simulink model "EEBL_Scenario_03_cs"  (Simulink 7.6)
settings: Solver=ode5  SolverMode=SingleTasking  StartTime=0.0  StopTime=15  FixedStep=1/100  RelTol=1e-3
PreLoadFcn:
  | check_NUTS_defined;
  | 
  | assignin('base',['model_closed_' bdroot],false);addpath('../includes_V2x');
InitFcn:
  | PreScanExperimentInitFcn(bdroot)
StopFcn:
  | PreScanExperimentStopFcn(bdroot)
undefined symbols (not defined in the file): acceleration, actorID, actorType, DiscIntNeverNeededParam, GPS_alt, GPS_lat, GPS_long, intmax, lightBarInUse, messageID, publicVehicleType, rotZ, sireneInUse, trafficLightPriority, turnAdvice, velocity, x_ini_VRML, y_ini_VRML, yawRate, z_ini_VRML
libraries: simulink x68, PreScanSimulinkLibrary x15, simulink_extras x9, PreScanUsefulBlocks x8, simulink_need_slupdate x1
(part 9 of 12)

== system EEBL_Scenario_03_cs/Audi_A8_1/Dynamics_Simple/ShiftLogic ==
  Throttle_[%] : Inport
  GearNr_[-] : Inport  Port=2
  Auto_GearShift : Inport  Port=3
  VehSpeed_[ms-1] : Inport  Port=4
  Add2 : Sum
  Data Type Conversion1 : DataTypeConversion  OutDataTypeStr=double
  Detect Increase1 : simulink/Logic and Bit Operations/Detect Increase  SystemSampleTime=-1  vinit=0.0
  Detect Increase : Subsystem
  Gear limitation : Saturate  UpperLimit=p.maxGear  LowerLimit=1
  Gear limitation while shifting : Saturate  UpperLimit=p.maxGear  LowerLimit=1
  GearNeutral : Constant  Value=0
  GearReverse : Constant  Value=-1
  "IC, gear = 1" : Memory  X0=1  InheritSampleTime=on
  If Action Neutral : Subsystem  TreatAsAtomicUnit=on
  If Action Normal : Subsystem  TreatAsAtomicUnit=on
  If Action Reverse : Subsystem  TreatAsAtomicUnit=on
  Memory : Memory  InheritSampleTime=on
  Merge : Merge  Inputs=3
  Relational Operator : RelationalOperator  OutDataTypeStr=boolean
  Relational Operator1 : RelationalOperator  Operator=<=  OutDataTypeStr=boolean
  Shift_Down time : simulink/Discrete/Integer Delay  NumDelays=p.ShiftDown_fac  InputProcessing=Inherited  vinit=0.0  samptime=-1
  Shift_Up time : simulink/Discrete/Integer Delay  NumDelays=p.ShiftUp_fac  InputProcessing=Inherited  vinit=0.0  samptime=-1
  Sum : Sum  Inputs=+-
  interp_down : Lookup2D  RowIndex=p.downth  ColumnIndex=[1:p.maxGear]  Table=p.downtab  LookUpMeth=Interpolation-Use End Values  InputSameDT=on
  interp_up : Lookup2D  RowIndex=p.upth  ColumnIndex=[1:p.maxGear]  Table=p.uptab  LookUpMeth=Interpolation-Use End Values  InputSameDT=on
  reverse/neutral/normal gear : If  IfExpression=u1 == 0  ElseIfExpressions=u1 < 0
  to_ms-1 : Gain  Gain=1/3.6
  "to_ms-1 " : Gain  Gain=1/3.6
  GearNr : Outport
  wires:
  Auto_GearShift/1 -> reverse/neutral/normal gear/1
  "IC, gear = 1"/1 -> If Action Normal/1(In1)
  Merge/1 -> GearNr/1
  If Action Reverse/1(Out1) -> Merge/2
  If Action Neutral/1(Out1) -> Merge/1
  If Action Normal/1(Out1) -> Merge/3
  reverse/neutral/normal gear/3 -> If Action Normal/Action
  reverse/neutral/normal gear/1 -> If Action Neutral/Action
  reverse/neutral/normal gear/2 -> If Action Reverse/Action
  GearReverse/1 -> If Action Reverse/1(In1)
  GearNeutral/1 -> If Action Neutral/1(In1)
  Shift_Down time/1 -> Sum/2
  Shift_Up time/1 -> Sum/1
  Detect Increase/1(Out1) -> Shift_Up time/1
  Data Type Conversion1/1 -> Shift_Down time/1
  Detect Increase1/1 -> Data Type Conversion1/1
  Sum/1 -> Add2/1
  Memory/1 -> Add2/2  "GearNr_[-]"
  Add2/1 -> Gear limitation while shifting/1
  Gear limitation while shifting/1 -> "IC, gear = 1"/1, Memory/1  "GearNr_[-]"
  Throttle_[%]/1 -> interp_down/1, interp_up/1
  Relational Operator/1 -> Detect Increase/2(In2)
  Relational Operator1/1 -> Detect Increase1/1
  interp_down/1 -> "to_ms-1 "/1
  VehSpeed_[ms-1]/1 -> Relational Operator/1, Relational Operator1/1
  interp_up/1 -> to_ms-1/1
  Gear limitation/1 -> interp_down/2, interp_up/2, Detect Increase/1(GearNr_[-])
  GearNr_[-]/1 -> Gear limitation/1
  to_ms-1/1 -> Relational Operator/2
  "to_ms-1 "/1 -> Relational Operator1/2

== system EEBL_Scenario_03_cs/Audi_A8_1/Dynamics_Simple/Transmission ==
  nEngine_[rpm] : Inport
  GearNr_[-] : Inport  Port=2
  n_TransmissionOut_[rpm] : Inport  Port=3
  Torque_Converter : Subsystem
      mask Display: image(imread('TorqueConverter.png'));
  Transmission_Ratio : Subsystem
  Viscous coupling : Lookup  InputValues=[-5:0.1:5]*p.m/4  Table=p.m/4*tanh([-5:0.1:5])
  ImpellerTorque_[Nm] : Outport  InitialOutput=0
  TransmissionTorque_[Nm] : Outport  Port=2  InitialOutput=0
  wires:
  Torque_Converter/2(TurbineTorque_[Nm]) -> Viscous coupling/1  "Converter_Torque_[Nm]"
  Transmission_Ratio/2(nTransmissionIn_[rpm]) -> Torque_Converter/2(nTransmission_[rpm])
  nEngine_[rpm]/1 -> Torque_Converter/1(nEngine_[rpm])
  GearNr_[-]/1 -> Transmission_Ratio/2(GearNr_[-]), Torque_Converter/3(Gear nr)
  n_TransmissionOut_[rpm]/1 -> Transmission_Ratio/3(nTransmissionOut_[rpm])
  Torque_Converter/1(ImpellerTorque_[Nm]) -> ImpellerTorque_[Nm]/1
  Transmission_Ratio/1(tTransmissionOut_[Nm]) -> TransmissionTorque_[Nm]/1
  Viscous coupling/1 -> Transmission_Ratio/1(tTransmissionIn_[Nm])

== system EEBL_Scenario_03_cs/Audi_A8_1/EEB/vehicle CAM generator ==
  note: System creates continous signals based on CAM protocol
  CAM_warning_in : Inport
  CAM_messageID_in : Inport  Port=2
  CAM_vehicleID_in : Inport  Port=3
  CAM_vehicleType_in : Inport  Port=4
  CAM_publicVehicleType_in : Inport  Port=5
  CAM_lightBarInUse_in : Inport  Port=6
  CAM_sireneInUse_in : Inport  Port=7
  CAM_velocity_in : Inport  Port=8
  CAM_acceleration_in : Inport  Port=9
  CAM_yawRate_in : Inport  Port=10
  CAM_turnAdvice_in : Inport  Port=11
  CAM_trafficLightPriority_in : Inport  Port=12
  CAM_GPSlat_in : Inport  Port=13
  CAM_GPSlong_in : Inport  Port=14
  CAM_GPSalt_in : Inport  Port=15
  CAM_rotZ_in : Inport  Port=16
  NoMissedMessages : Inport  Port=17
  MessageDelay : Inport  Port=18
  CAM delay : Subsystem
  For Iterator Subsystem : Subsystem  TreatAsAtomicUnit=on
  Memory : Memory
  Memory1 : Memory
  Probe : Probe  ProbeWidth=off  ProbeSampleTime=off  ProbeComplexSignal=off  ProbeSignalDimensions=on
  Rounding Function1 : Rounding
  Seperate signals : Stateflow chart  TreatAsAtomicUnit=on
  Signal Matrix create : Stateflow chart  TreatAsAtomicUnit=on
  CAM_warning : Outport
  CAM_messageID : Outport  Port=2
  CAM_vehicleID : Outport  Port=3
  CAM_vehicleType : Outport  Port=4
  CAM_publicVehicleType : Outport  Port=5
  CAM_lightBarInUse : Outport  Port=6
  CAM_sireneInUse : Outport  Port=7
  CAM_velocity : Outport  Port=8
  CAM_acceleration : Outport  Port=9
  CAM_yawRate : Outport  Port=10
  CAM_turnAdvice : Outport  Port=11
  CAM_trafficLightPriority : Outport  Port=12
  CAM_GPSlat : Outport  Port=13
  CAM_GPSlong : Outport  Port=14
  CAM_GPSalt : Outport  Port=15
  CAM_rotZ : Outport  Port=16
  wires:
  Seperate signals/16(CAM_rotZ) -> CAM_rotZ/1
  Seperate signals/15(CAM_GPSalt) -> CAM_GPSalt/1
  Seperate signals/14(CAM_GPSlong) -> CAM_GPSlong/1
  Seperate signals/13(CAM_GPSlat) -> CAM_GPSlat/1
  Seperate signals/12(CAM_trafficLightPriority) -> CAM_trafficLightPriority/1
  Seperate signals/11(CAM_turnAdvice) -> CAM_turnAdvice/1
  Seperate signals/10(CAM_yawRate) -> CAM_yawRate/1
  Seperate signals/9(CAM_acceleration) -> CAM_acceleration/1
  Seperate signals/8(CAM_velocity) -> CAM_velocity/1
  Seperate signals/7(CAM_sireneInUse) -> CAM_sireneInUse/1
  Seperate signals/6(CAM_lightBarInUse) -> CAM_lightBarInUse/1
  Seperate signals/5(CAM_publicVehicleType) -> CAM_publicVehicleType/1
  Seperate signals/4(CAM_vehicleType) -> CAM_vehicleType/1
  Seperate signals/3(CAM_vehicleID) -> CAM_vehicleID/1
  Seperate signals/2(CAM_messageID) -> CAM_messageID/1
  Seperate signals/1(CAM_warning) -> CAM_warning/1
  CAM_warning_in/1 -> Signal Matrix create/1(CAM_warning)
  CAM_messageID_in/1 -> Signal Matrix create/2(CAM_messageID)
  CAM_vehicleID_in/1 -> Signal Matrix create/3(CAM_vehicleID), Probe/1
  CAM_vehicleType_in/1 -> Signal Matrix create/4(CAM_vehicleType)
  CAM_publicVehicleType_in/1 -> Signal Matrix create/5(CAM_publicVehicleType)
  CAM_lightBarInUse_in/1 -> Signal Matrix create/6(CAM_lightBarInUse)
  CAM_sireneInUse_in/1 -> Signal Matrix create/7(CAM_sireneInUse)
  CAM_velocity_in/1 -> Signal Matrix create/8(CAM_velocity)
  CAM_acceleration_in/1 -> Signal Matrix create/9(CAM_acceleration)
  CAM_yawRate_in/1 -> Signal Matrix create/10(CAM_yawRate)
  CAM_turnAdvice_in/1 -> Signal Matrix create/11(CAM_turnAdvice)
  CAM_trafficLightPriority_in/1 -> Signal Matrix create/12(CAM_trafficLightPriority)
  CAM_GPSlat_in/1 -> Signal Matrix create/13(CAM_GPSlat)
  CAM_GPSlong_in/1 -> Signal Matrix create/14(CAM_GPSlong)
  CAM_GPSalt_in/1 -> Signal Matrix create/15(CAM_GPSalt)
  CAM_rotZ_in/1 -> Signal Matrix create/16(CAM_rotZ)
  Memory/1 -> For Iterator Subsystem/3(CAM_old)
  For Iterator Subsystem/1(CAM_o) -> Memory/1, Seperate signals/1(CAM)
  Probe/1 -> For Iterator Subsystem/2(Size)
  Signal Matrix create/1(CAM) -> CAM delay/1(in)
  MessageDelay/1 -> CAM delay/2(Tdelay)
  CAM delay/1(out) -> For Iterator Subsystem/1(CAM_in)
  For Iterator Subsystem/2(tmp_out) -> Memory1/1
  Memory1/1 -> For Iterator Subsystem/5(tmp_in)
  NoMissedMessages/1 -> Rounding Function1/1
  Rounding Function1/1 -> For Iterator Subsystem/4(NoMM)

== system EEBL_Scenario_03_cs/Audi_A8_1/PathFollower_1/CTRL REFERENCES ==
  note: REFERENCE POSITION BASED POSITION CTRL
  Pos x,y,Y [m,m,rad] : Inport
  Position Preview Distance [m] : Inport  Port=2
  TrajOffset [m,m,rad] : Inport  Port=3
  ActorOffset_Left(+) / Right(-)_[m] : Inport  Port=4
  Calculate Preview Point (pvp) by extrapolating current Vehicle Position (p0) with Preview Distance and Vehicle Orientation : Subsystem
  Find Reference Point (pref)  on Trajectory closest  to PreView Point (pvp) : M-S-Function  FunctionName=msfcn_find_closest_trajectory_points  Parameters=[Traj_x Traj_y]
      mask Display:
      | port_label('input', 1, 'pvp')
      | port_label('input', 2, 'TrajOffset_x_y_Y')
      | port_label('input', 3, 'ActorOffset_Left+/Right-')
      | port_label('input', 4, 'p0')
      | port_label('output', 1, 'pref')
  Find Reference Point (pref0)  on Trajectory closest  to P0 Point (p0) : M-S-Function  FunctionName=msfcn_find_closest_trajectory_points0  Parameters=[Traj_x Traj_y]
      mask Display:
      | port_label('input', 1, 'pvp')
      | port_label('input', 2, 'TrajOffset_x_y_Y')
      | port_label('input', 3, 'ActorOffset_Left+/Right-')
      | port_label('input', 4, 'p0')
      | port_label('output', 1, 'pref_0')
      | port_label('output', 2, 'Actor/Traj_distance')
      | port_label('output', 3, 'Actor/Traj_angle')
  Mux1 : Mux  Inputs=2
  Selector1 : Selector  InputPortWidth=3  IndexOptions=Index vector (dialog)  Indices=[1 2]  OutputSizes=1
  Terminator : Terminator
  pvp  [m,m] : Outport
  pref_pvp [m,m] : Outport  Port=2
  pref_0 [m,m] : Outport  Port=3
  Actor/Traj_distance [m] : Outport  Port=4
  Actor/Traj_angle [deg] : Outport  Port=5
  wires:
  Mux1/1 -> pvp  [m,m]/1, Find Reference Point (pref)  on Trajectory closest  to PreView Point (pvp)/1, Find Reference Point (pref0)  on Trajectory closest  to P0 Point (p0)/1
  Pos x,y,Y [m,m,rad]/1 -> Calculate Preview Point (pvp) by extrapolating current Vehicle Position (p0) with Preview Distance and Vehicle Orientation/2(x,y,Y Demux [m,m,rad]), Find Reference Point (pref0)  on Trajectory closest  to P0 Point (p0)/4, Selector1/1
  Calculate Preview Point (pvp) by extrapolating current Vehicle Position (p0) with Preview Distance and Vehicle Orientation/1(x_glob_PVD) -> Mux1/1
  Calculate Preview Point (pvp) by extrapolating current Vehicle Position (p0) with Preview Distance and Vehicle Orientation/3(Y [rad]) -> Terminator/1
  Position Preview Distance [m]/1 -> Calculate Preview Point (pvp) by extrapolating current Vehicle Position (p0) with Preview Distance and Vehicle Orientation/1(Preview Distance)
  Find Reference Point (pref)  on Trajectory closest  to PreView Point (pvp)/1 -> pref_pvp [m,m]/1
  Find Reference Point (pref0)  on Trajectory closest  to P0 Point (p0)/1 -> pref_0 [m,m]/1
  Calculate Preview Point (pvp) by extrapolating current Vehicle Position (p0) with Preview Distance and Vehicle Orientation/2(y_glob_PVD) -> Mux1/2
  TrajOffset [m,m,rad]/1 -> Find Reference Point (pref)  on Trajectory closest  to PreView Point (pvp)/2, Find Reference Point (pref0)  on Trajectory closest  to P0 Point (p0)/2  "L6"
  ActorOffset_Left(+) / Right(-)_[m]/1 -> Find Reference Point (pref)  on Trajectory closest  to PreView Point (pvp)/3, Find Reference Point (pref0)  on Trajectory closest  to P0 Point (p0)/3
  Selector1/1 -> Find Reference Point (pref)  on Trajectory closest  to PreView Point (pvp)/4
  Find Reference Point (pref0)  on Trajectory closest  to P0 Point (p0)/2 -> Actor/Traj_distance [m]/1
  Find Reference Point (pref0)  on Trajectory closest  to P0 Point (p0)/3 -> Actor/Traj_angle [deg]/1

== system EEBL_Scenario_03_cs/Audi_A8_1/PathFollower_1/Calculate shifted p0 wrt COG ==
  position x,y,Y [m,m,deg] : Inport
  Constant1 : Constant  Value=XShifting_wrt_COG
  Degrees to Radians : simulink_extras/Transformations/Degrees to Radians  SystemSampleTime=-1
  Demux1 : Demux  Outputs=3
  Fcn : Fcn  Expr=u(2)*cos(u(1))
  Fcn1 : Fcn  Expr=u(2)*sin(u(1))
  Mux1 : Mux  Inputs=3
  Mux2 : Mux  Inputs=2
  Sum : Sum  Inputs=|++
  Sum1 : Sum  Inputs=|++
  position x,y,Y [m,m,rad] : Outport
  wires:
  Sum/1 -> Mux1/1
  Sum1/1 -> Mux1/2
  Demux1/1 -> Sum/1
  Demux1/3 -> Degrees to Radians/1
  Degrees to Radians/1 -> Mux2/1, Mux1/3
  Mux2/1 -> Fcn/1, Fcn1/1
  Fcn/1 -> Sum/2
  Fcn1/1 -> Sum1/2
  Demux1/2 -> Sum1/1
  position x,y,Y [m,m,deg]/1 -> Demux1/1
  Mux1/1 -> position x,y,Y [m,m,rad]/1
  Constant1/1 -> Mux2/2

== system EEBL_Scenario_03_cs/Audi_A8_1/PathFollower_1/DELTA CTRL ==
  note: POSITION BASED STEERWHEEL CONTROL
  p0 : Inport
  pvp : Inport  Port=2
  pref_pvp : Inport  Port=3
  pref0 : Inport  Port=4
  Calculate  preview angle : M-S-Function  FunctionName=msfcn_preview_angle_and_distance
      mask Display:
      | port_label('input', 2, 'pref [m,m]')
      | port_label('input', 3, 'p0 [m,m]')
      | port_label('input', 1, 'pvp [m,m]')
      | 
      | port_label('output', 1, 'angle [rad]')
  Divide2 : Product
  Divide4 : Product
  Error check : Subsystem
  Goto Tag Visibility : GotoTagVisibility  GotoTag=pref0
  Goto Tag Visibility1 : GotoTagVisibility  GotoTag=p0
  Radians to Degrees1 : simulink_extras/Transformations/Radians to Degrees  SystemSampleTime=-1
  Selector2 : Selector  InputPortWidth=3  IndexOptions=Index vector (dialog)  Indices=[1 2]  OutputSizes=1
  Steering angle  velocity dependent : Lookup  InputValues=[0 18 40 60 70 80 90 100 110]  Table=[16.5 16.5 28 44.5 55 60.5 60.5 60.5 60.5]
  Steering angle preview  distance dependent : Lookup  InputValues=[0 1 4 5 6 7 8 9 10 11 20 21]  Table=[1.5 1.5 1 1 1 1 1 1 0.9 0.9 0.8 0.8]
  These limits are  the vehicle maximum  steering wheel angle : Saturate  UpperLimit=720  LowerLimit=-720
  TunableSteering Gain : Gain  Gain=TunableSteeringGain
  sign1 : Gain  Gain=3.6
  delta_steerwheel [deg] : Outport
  tag scope: p0=scoped, pref0=scoped
  wires:
  Calculate  preview angle/1 -> Radians to Degrees1/1
  Selector2/1 -> Calculate  preview angle/3
  p0/1 -> Selector2/1, [p0]
  pvp/1 -> Calculate  preview angle/1
  pref_pvp/1 -> Calculate  preview angle/2
  Radians to Degrees1/1 -> Divide2/2
  These limits are  the vehicle maximum  steering wheel angle/1 -> delta_steerwheel [deg]/1
  pref0/1 -> [pref0]
  sign1/1 -> Steering angle  velocity dependent/1
  [v_actual] -> sign1/1
  Steering angle  velocity dependent/1 -> Divide2/1
  Divide4/1 -> TunableSteering Gain/1
  Divide2/1 -> Divide4/1
  Steering angle preview  distance dependent/1 -> Divide4/2
  [PreviewDistance] -> Steering angle preview  distance dependent/1
  TunableSteering Gain/1 -> These limits are  the vehicle maximum  steering wheel angle/1

== system EEBL_Scenario_03_cs/Audi_A8_1/PathFollower_1/THROTTLE CTRL ==
  v_actual [m/s] : Inport
  Desired Velocity [m/s] : Inport  Port=2
  Initial Velocity [m/s] : Inport  Port=3
  Demux : Demux  Outputs=3
  GearNormal : Constant
  "GearNormal " : Constant
  If Desired Velocity = 0 : Subsystem  TreatAsAtomicUnit=on
  If Desired Velocity ~= 0 : Subsystem  TreatAsAtomicUnit=on
  Merge : Merge
  Mux : Mux  Inputs=3
  Mux2 : Mux  Inputs=3
  Sum4 : Sum  Inputs=|+-
  if : If  IfExpression=u1 == 0
  throttle [%] : Outport
  brake pressure [bar] : Outport  Port=2
  v0 [m/s] : Outport  Port=3
  Auto_GearShift : Outport  Port=4
  wires:
  v_actual [m/s]/1 -> Sum4/2
  If Desired Velocity ~= 0/3(Auto_GearShift) -> Mux2/3
  If Desired Velocity ~= 0/2(brake pressure [bar]) -> Mux2/2
  If Desired Velocity ~= 0/1(throttle [%]) -> Mux2/1
  if/1 -> If Desired Velocity = 0/Action
  if/2 -> If Desired Velocity ~= 0/Action
  If Desired Velocity = 0/3(Auto_GearShift) -> Mux/3
  "GearNormal "/1 -> If Desired Velocity ~= 0/1(In1)
  Demux/3 -> Auto_GearShift/1
  Demux/2 -> brake pressure [bar]/1
  Demux/1 -> throttle [%]/1
  Mux/1 -> Merge/1
  Mux2/1 -> Merge/2
  If Desired Velocity = 0/2(brake pressure [bar]) -> Mux/2
  If Desired Velocity = 0/1(throttle [%]) -> Mux/1
  Merge/1 -> Demux/1
  GearNormal/1 -> If Desired Velocity = 0/1(In1)
  Initial Velocity [m/s]/1 -> v0 [m/s]/1
  Desired Velocity [m/s]/1 -> Sum4/1, if/1
  Sum4/1 -> If Desired Velocity ~= 0/2(Desired Velocity [m/s])

== system EEBL_Scenario_03_cs/Audi_A8_1/SELF_Demux/compas converter ==
  rotz [rad] : Inport
  cart2compas : Subsystem
  rad2deg : Gain  Gain=180/pi
  heading [deg] : Outport
  wires:
  cart2compas/1(heading [deg]) -> heading [deg]/1
  rotz [rad]/1 -> rad2deg/1
  rad2deg/1 -> cart2compas/1(Angle [deg])

== system EEBL_Scenario_03_cs/Audi_A8_1/Trajectories/Traj2State1 ==
  Traj Org : Inport
  Offset : Inport  Port=2
  Add2 : Sum
  ApplyRotation : PreScanSimulinkLibrary/ApplyRotation  SystemSampleTime=-1
  ApplyRotation1 : PreScanSimulinkLibrary/ApplyRotation  SystemSampleTime=-1
  ApplyRotation2 : PreScanSimulinkLibrary/ApplyRotation  SystemSampleTime=-1
  Constant : Constant  Value=zeros(12,1)
  Mux : Mux  Inputs=6
  Mux1 : Mux  Inputs=2
  Mux{2,4..9} (7 alike) : Mux  Inputs=3
  Mux3 : Mux  Inputs=2
  Selector : Selector  InputPortWidth=6  IndexOptions=Index vector (dialog)  Indices=[4 5 6]  OutputSizes=1
  Selector1 : Selector  InputPortWidth=21  IndexOptions=Index vector (dialog)  Indices=[5]  OutputSizes=1
  Selector10 : Selector  InputPortWidth=21  IndexOptions=Index vector (dialog)  Indices=[2]  OutputSizes=1
  Selector11 : Selector  InputPortWidth=21  IndexOptions=Index vector (dialog)  Indices=[3]  OutputSizes=1
  Selector12 : Selector  InputPortWidth=21  IndexOptions=Index vector (dialog)  Indices=[1]  OutputSizes=1
  Selector13 : Selector  InputPortWidth=21  IndexOptions=Index vector (dialog)  Indices=[8]  OutputSizes=1
  Selector14 : Selector  InputPortWidth=21  IndexOptions=Index vector (dialog)  Indices=[9]  OutputSizes=1
  Selector15 : Selector  InputPortWidth=21  IndexOptions=Index vector (dialog)  Indices=[7]  OutputSizes=1
  Selector16 : Selector  InputPortWidth=21  IndexOptions=Index vector (dialog)  Indices=[14]  OutputSizes=1
  Selector17 : Selector  InputPortWidth=21  IndexOptions=Index vector (dialog)  Indices=[15]  OutputSizes=1
  Selector18 : Selector  InputPortWidth=21  IndexOptions=Index vector (dialog)  Indices=[13]  OutputSizes=1
  Selector19 : Selector  InputPortWidth=21  IndexOptions=Index vector (dialog)  Indices=[20]  OutputSizes=1
  Selector2 : Selector  InputPortWidth=21  IndexOptions=Index vector (dialog)  Indices=[6]  OutputSizes=1
  Selector20 : Selector  InputPortWidth=21  IndexOptions=Index vector (dialog)  Indices=[21]  OutputSizes=1
  Selector21 : Selector  InputPortWidth=21  IndexOptions=Index vector (dialog)  Indices=[19]  OutputSizes=1
  Selector3 : Selector  InputPortWidth=21  IndexOptions=Index vector (dialog)  Indices=[12]  OutputSizes=1
  Selector4 : Selector  InputPortWidth=21  IndexOptions=Index vector (dialog)  Indices=[17]  OutputSizes=1
  Selector5 : Selector  InputPortWidth=21  IndexOptions=Index vector (dialog)  Indices=[18]  OutputSizes=1
  Selector6 : Selector  InputPortWidth=21  IndexOptions=Index vector (dialog)  Indices=[16]  OutputSizes=1
  Selector7 : Selector  InputPortWidth=21  IndexOptions=Index vector (dialog)  Indices=[11]  OutputSizes=1
  Selector8 : Selector  InputPortWidth=21  IndexOptions=Index vector (dialog)  Indices=[10]  OutputSizes=1
  Selector9 : Selector  InputPortWidth=21  IndexOptions=Index vector (dialog)  Indices=[4]  OutputSizes=1
  Traj2State2 : Subsystem
  state : Outport
  wires:
  Mux9/1 -> ApplyRotation2/2, ApplyRotation1/2, ApplyRotation/2
  Selector20/1 -> Mux9/3
  Selector19/1 -> Mux9/2
  Selector21/1 -> Mux9/1
  Selector5/1 -> Mux8/3
  Selector4/1 -> Mux8/2
  Selector6/1 -> Mux8/1
  Mux8/1 -> Mux/6
  Mux6/1 -> ApplyRotation2/1
  Mux7/1 -> Mux/4
  ApplyRotation2/1 -> Mux/5
  Selector3/1 -> Mux7/3
  Selector7/1 -> Mux7/2
  Selector8/1 -> Mux7/1
  Mux4/1 -> Mux/2
  Mux5/1 -> ApplyRotation1/1
  ApplyRotation1/1 -> Mux/3
  Mux2/1 -> ApplyRotation/1
  ApplyRotation/1 -> Mux/1
  Selector2/1 -> Mux4/3
  Selector1/1 -> Mux4/2
  Selector9/1 -> Mux4/1
  Selector17/1 -> Mux6/3
  Selector16/1 -> Mux6/2
  Selector18/1 -> Mux6/1
  Selector14/1 -> Mux5/3
  Selector13/1 -> Mux5/2
  Selector15/1 -> Mux5/1
  Selector11/1 -> Mux2/3
  Selector10/1 -> Mux2/2
  Selector12/1 -> Mux2/1
  Mux3/1 -> Selector8/1, Selector7/1, Selector3/1, Selector18/1, Selector16/1, Selector17/1, Selector6/1, Selector20/1, Selector19/1, Selector21/1, Selector5/1, Selector4/1, Selector14/1, Selector13/1, Selector15/1, Selector2/1, Selector1/1, Selector9/1, Selector12/1, Selector10/1, Selector11/1
  Mux1/1 -> Add2/2
  Constant/1 -> Mux1/2
  Add2/1 -> Traj2State2/1(traj)
  Selector/1 -> Mux3/2
  Traj Org/1 -> Mux3/1
  Offset/1 -> Mux1/1, Selector/1
  Mux/1 -> Add2/1
  Traj2State2/1(state) -> state/1

== system EEBL_Scenario_03_cs/Audi_A8_1/Trajectories/Trajectory_1 ==
  From Workspace : FromWorkspace  VariableName=trajectory  SampleTime=TimeStep  OutputAfterFinalValue=Holding final value
  From Workspace1 : FromWorkspace  VariableName=trajectory  SampleTime=TimeStep  OutputAfterFinalValue=Setting to zero
  Mux : Mux  Inputs=2
  Selector1 : Selector  InputPortWidth=24  IndexOptions=Index vector (dialog)  Indices=[7:18]  OutputSizes=1
  Selector9 : Selector  InputPortWidth=24  IndexOptions=Index vector (dialog)  Indices=[1:6]  OutputSizes=1
  trajectory : Outport
  wires:
  Selector1/1 -> Mux/2
  Selector9/1 -> Mux/1
  Mux/1 -> trajectory/1
  From Workspace1/1 -> Selector1/1
  From Workspace/1 -> Selector9/1

== system EEBL_Scenario_03_cs/BMW_X5_1/Antenna_Rx_3_Demux/Reorder ==
  In : Inport
  Selector1 : Selector  InputPortWidth=InputPortWidth  IndexOptions=Index vector (dialog)  Indices=Elements  OutputSizes=1
  Out : Outport
  wires:
  Selector1/1 -> Out/1
  In/1 -> Selector1/1

== system EEBL_Scenario_03_cs/BMW_X5_1/Antenna_Rx_3_Demux/compas converter ==
  rotz [rad] : Inport
  cart2compas : Subsystem
  rad2deg : Gain  Gain=180/pi
  heading [deg] : Outport
  wires:
  rad2deg/1 -> cart2compas/1(Angle [deg])
  rotz [rad]/1 -> rad2deg/1
  cart2compas/1(heading [deg]) -> heading [deg]/1

== system EEBL_Scenario_03_cs/BMW_X5_1/SELF_Demux/compas converter ==
  rotz [rad] : Inport
  cart2compas : Subsystem
  rad2deg : Gain  Gain=180/pi
  heading [deg] : Outport
  wires:
  cart2compas/1(heading [deg]) -> heading [deg]/1
  rotz [rad]/1 -> rad2deg/1
  rad2deg/1 -> cart2compas/1(Angle [deg])

== system EEBL_Scenario_03_cs/BMW_X5_1/Trajectories/Traj2State1 ==
  Traj Org : Inport
  Offset : Inport  Port=2
  Add2 : Sum
  ApplyRotation : PreScanSimulinkLibrary/ApplyRotation  SystemSampleTime=-1
  ApplyRotation1 : PreScanSimulinkLibrary/ApplyRotation  SystemSampleTime=-1
  ApplyRotation2 : PreScanSimulinkLibrary/ApplyRotation  SystemSampleTime=-1
  Constant : Constant  Value=zeros(12,1)
  Mux : Mux  Inputs=6
  Mux1 : Mux  Inputs=2
  Mux{2,4..9} (7 alike) : Mux  Inputs=3
  Mux3 : Mux  Inputs=2
  Selector : Selector  InputPortWidth=6  IndexOptions=Index vector (dialog)  Indices=[4 5 6]  OutputSizes=1
  Selector1 : Selector  InputPortWidth=21  IndexOptions=Index vector (dialog)  Indices=[5]  OutputSizes=1
  Selector10 : Selector  InputPortWidth=21  IndexOptions=Index vector (dialog)  Indices=[2]  OutputSizes=1
  Selector11 : Selector  InputPortWidth=21  IndexOptions=Index vector (dialog)  Indices=[3]  OutputSizes=1
  Selector12 : Selector  InputPortWidth=21  IndexOptions=Index vector (dialog)  Indices=[1]  OutputSizes=1
  Selector13 : Selector  InputPortWidth=21  IndexOptions=Index vector (dialog)  Indices=[8]  OutputSizes=1
  Selector14 : Selector  InputPortWidth=21  IndexOptions=Index vector (dialog)  Indices=[9]  OutputSizes=1
  Selector15 : Selector  InputPortWidth=21  IndexOptions=Index vector (dialog)  Indices=[7]  OutputSizes=1
  Selector16 : Selector  InputPortWidth=21  IndexOptions=Index vector (dialog)  Indices=[14]  OutputSizes=1
  Selector17 : Selector  InputPortWidth=21  IndexOptions=Index vector (dialog)  Indices=[15]  OutputSizes=1
  Selector18 : Selector  InputPortWidth=21  IndexOptions=Index vector (dialog)  Indices=[13]  OutputSizes=1
  Selector19 : Selector  InputPortWidth=21  IndexOptions=Index vector (dialog)  Indices=[20]  OutputSizes=1
  Selector2 : Selector  InputPortWidth=21  IndexOptions=Index vector (dialog)  Indices=[6]  OutputSizes=1
  Selector20 : Selector  InputPortWidth=21  IndexOptions=Index vector (dialog)  Indices=[21]  OutputSizes=1
  Selector21 : Selector  InputPortWidth=21  IndexOptions=Index vector (dialog)  Indices=[19]  OutputSizes=1
  Selector3 : Selector  InputPortWidth=21  IndexOptions=Index vector (dialog)  Indices=[12]  OutputSizes=1
  Selector4 : Selector  InputPortWidth=21  IndexOptions=Index vector (dialog)  Indices=[17]  OutputSizes=1
  Selector5 : Selector  InputPortWidth=21  IndexOptions=Index vector (dialog)  Indices=[18]  OutputSizes=1
  Selector6 : Selector  InputPortWidth=21  IndexOptions=Index vector (dialog)  Indices=[16]  OutputSizes=1
  Selector7 : Selector  InputPortWidth=21  IndexOptions=Index vector (dialog)  Indices=[11]  OutputSizes=1
  Selector8 : Selector  InputPortWidth=21  IndexOptions=Index vector (dialog)  Indices=[10]  OutputSizes=1
  Selector9 : Selector  InputPortWidth=21  IndexOptions=Index vector (dialog)  Indices=[4]  OutputSizes=1
  Traj2State2 : Subsystem
  state : Outport
  wires:
  Mux9/1 -> ApplyRotation2/2, ApplyRotation1/2, ApplyRotation/2
  Selector20/1 -> Mux9/3
  Selector19/1 -> Mux9/2
  Selector21/1 -> Mux9/1
  Selector5/1 -> Mux8/3
  Selector4/1 -> Mux8/2
  Selector6/1 -> Mux8/1
  Mux8/1 -> Mux/6
  Mux6/1 -> ApplyRotation2/1
  Mux7/1 -> Mux/4
  ApplyRotation2/1 -> Mux/5
  Selector3/1 -> Mux7/3
  Selector7/1 -> Mux7/2
  Selector8/1 -> Mux7/1
  Mux4/1 -> Mux/2
  Mux5/1 -> ApplyRotation1/1
  ApplyRotation1/1 -> Mux/3
  Mux2/1 -> ApplyRotation/1
  ApplyRotation/1 -> Mux/1
  Selector2/1 -> Mux4/3
  Selector1/1 -> Mux4/2
  Selector9/1 -> Mux4/1
  Selector17/1 -> Mux6/3
  Selector16/1 -> Mux6/2
  Selector18/1 -> Mux6/1
  Selector14/1 -> Mux5/3
  Selector13/1 -> Mux5/2
  Selector15/1 -> Mux5/1
  Selector11/1 -> Mux2/3
  Selector10/1 -> Mux2/2
  Selector12/1 -> Mux2/1
  Mux3/1 -> Selector8/1, Selector7/1, Selector3/1, Selector18/1, Selector16/1, Selector17/1, Selector6/1, Selector20/1, Selector19/1, Selector21/1, Selector5/1, Selector4/1, Selector14/1, Selector13/1, Selector15/1, Selector2/1, Selector1/1, Selector9/1, Selector12/1, Selector10/1, Selector11/1
  Mux1/1 -> Add2/2
  Constant/1 -> Mux1/2
  Add2/1 -> Traj2State2/1(traj)
  Selector/1 -> Mux3/2
  Traj Org/1 -> Mux3/1
  Offset/1 -> Mux1/1, Selector/1
  Mux/1 -> Add2/1
  Traj2State2/1(state) -> state/1

== system EEBL_Scenario_03_cs/BMW_X5_1/Trajectories/Trajectory_2 ==
  From Workspace : FromWorkspace  VariableName=trajectory  SampleTime=TimeStep  OutputAfterFinalValue=Holding final value
  From Workspace1 : FromWorkspace  VariableName=trajectory  SampleTime=TimeStep  OutputAfterFinalValue=Setting to zero
  Mux : Mux  Inputs=2
  Selector1 : Selector  InputPortWidth=24  IndexOptions=Index vector (dialog)  Indices=[7:18]  OutputSizes=1
  Selector9 : Selector  InputPortWidth=24  IndexOptions=Index vector (dialog)  Indices=[1:6]  OutputSizes=1
  trajectory : Outport
  wires:
  Selector1/1 -> Mux/2
  Selector9/1 -> Mux/1
  Mux/1 -> trajectory/1
  From Workspace1/1 -> Selector1/1
  From Workspace/1 -> Selector9/1

== system EEBL_Scenario_03_cs/BMW_X5_1/vehicle CAM generator/CAM generation ==
  x [m] : Inport
  y [m] : Inport  Port=2
  z [m] : Inport  Port=3
  rotZ [deg] : Inport  Port=4
  velocity [m/s] : Inport  Port=5
  Enable : EnablePort  StatesWhenEnabling=reset  PropagateVarSize=During execution
  Add : Sum  Inputs=+-
  Data Store Memory : DataStoreMemory  DataStoreName=CAM_time
  Data Store Memory1 : DataStoreMemory  DataStoreName=CAM_velocity
  Data Store Memory2 : DataStoreMemory  DataStoreName=CAM_heading
  Data Store Memory3 : DataStoreMemory  DataStoreName=CAM_x
  Data Store Memory4 : DataStoreMemory  DataStoreName=CAM_y
  Data Store Memory5 : DataStoreMemory  DataStoreName=CAM_z
  Data Store Read : DataStoreRead  DataStoreName=CAM_time  SampleTime=0.01
  Digital Clock : DigitalClock  SampleTime=0.01
  Merge : Merge  Inputs=3
  if : If  IfExpression=u1 >= 1  ElseIfExpressions=u1 < 0.1
  maybe : Subsystem  TreatAsAtomicUnit=on
  no : Subsystem  TreatAsAtomicUnit=on
  yes : Subsystem  TreatAsAtomicUnit=on
  CAN generation signal : Outport  OutputWhenDisabled=reset  InitialOutput=0
  wires:
  Digital Clock/1 -> Add/1
  Data Store Read/1 -> Add/2
  Add/1 -> if/1
  if/1 -> yes/Action
  yes/1(Out1) -> Merge/1
  no/1(Out1) -> Merge/2
  if/2 -> no/Action
  if/3 -> maybe/Action
  Merge/1 -> CAN generation signal/1
  x [m]/1 -> maybe/1(x [m]), yes/1(x [m])
  y [m]/1 -> maybe/2(y [m]), yes/2(y [m])
  z [m]/1 -> maybe/3(z [m]), yes/3(z [m])
  rotZ [deg]/1 -> maybe/4(rotZ [deg]), yes/4(rotZ [deg])
  velocity [m/s]/1 -> maybe/5(velocity [m/s]), yes/5(velocity [m/s])
  maybe/1(Out1) -> Merge/3

== system EEBL_Scenario_03_cs/BMW_X5_1/vehicle CAM generator/Enabled Subsystem ==
  CAM_sig : Inport
  Enable : EnablePort  PropagateVarSize=During execution
  CAM_signals : Outport  OutputWhenDisabled=reset  InitialOutput=0
  wires:
  CAM_sig/1 -> CAM_signals/1

== system EEBL_Scenario_03_cs/BMW_X5_1/vehicle CAM generator/Subsystem ==
  In1 : Inport
  GPS_Noise_src : Inport  Port=2
  GPS Noise : Subsystem
  Sum2 : Sum  Inputs=|++
  Out1 : Outport
  wires:
  GPS Noise/1(GPS_Noise) -> Sum2/2
  In1/1 -> Sum2/1
  Sum2/1 -> Out1/1
  GPS_Noise_src/1 -> GPS Noise/1(GPS_Noise_src)

== system EEBL_Scenario_03_cs/BMW_X5_1/vehicle CAM generator/Subsystem1 ==
  In1 : Inport
  GPS_Noise_src : Inport  Port=2
  GPS Noise : Subsystem
  Sum2 : Sum  Inputs=|++
  Out1 : Outport
  wires:
  GPS_Noise_src/1 -> GPS Noise/1(GPS_Noise_src)
  Sum2/1 -> Out1/1
  In1/1 -> Sum2/1
  GPS Noise/1(GPS_Noise) -> Sum2/2

== system EEBL_Scenario_03_cs/BMW_X5_1/vehicle CAM generator/Subsystem2 ==
  In1 : Inport
  GPS_Noise_src : Inport  Port=2
  GPS Noise : Subsystem
  Sum2 : Sum  Inputs=|++
  Out1 : Outport
  wires:
  GPS Noise/1(GPS_Noise) -> Sum2/2
  In1/1 -> Sum2/1
  Sum2/1 -> Out1/1
  GPS_Noise_src/1 -> GPS Noise/1(GPS_Noise_src)

== system EEBL_Scenario_03_cs/BMW_X5_1/vehicle CAM generator/Subsystem3 ==
  In1 : Inport
  GPS_Noise_src : Inport  Port=2
  GPS Noise : Subsystem
  Sum2 : Sum  Inputs=|++
  Out1 : Outport
  wires:
  GPS_Noise_src/1 -> GPS Noise/1(GPS_Noise_src)
  Sum2/1 -> Out1/1
  In1/1 -> Sum2/1
  GPS Noise/1(GPS_Noise) -> Sum2/2

== system EEBL_Scenario_03_cs/BMW_X5_1/vehicle CAM generator/impulse generator ==
  CAM_time_step : Inport
  Add : Sum
  Compare To Zero : simulink/Logic and Bit Operations/Compare To Zero  SystemSampleTime=-1  relop=>  LogicOutDataTypeMode=boolean  ZeroCross=off
  Data Type Conversion : DataTypeConversion  OutDataTypeStr=boolean
  Detect Change : simulink/Logic and Bit Operations/Detect Change  SystemSampleTime=-1  vinit=0
  Digital Clock1 : DigitalClock  SampleTime=0.01
  Divide : Product  Inputs=*/
  Gain : Gain  Gain=pi
  Product : Product  RndMeth=Zero
  Trigonometric Function : Trigonometry
  constant : Constant
  experiment time step : Constant  Value=0.01  SampleTime=0
  enable : Outport
  wires:
  Digital Clock1/1 -> Product/1
  Gain/1 -> Product/2
  Trigonometric Function/1 -> Compare To Zero/1
  Compare To Zero/1 -> Detect Change/1
  Detect Change/1 -> Data Type Conversion/1
  Product/1 -> Add/1
  constant/1 -> Divide/1
  Divide/1 -> Gain/1
  Add/1 -> Trigonometric Function/1
  experiment time step/1 -> Add/2
  Data Type Conversion/1 -> enable/1
  CAM_time_step/1 -> Divide/2

== system EEBL_Scenario_03_cs/BMW_X5_1/vehicle CAM generator/impulse generator1 ==
  CAM_time_step : Inport
  Add : Sum
  Compare To Zero : simulink/Logic and Bit Operations/Compare To Zero  SystemSampleTime=-1  relop=>  LogicOutDataTypeMode=boolean  ZeroCross=off
  Data Type Conversion : DataTypeConversion  OutDataTypeStr=boolean
  Detect Change : simulink/Logic and Bit Operations/Detect Change  SystemSampleTime=-1  vinit=0
  Digital Clock1 : DigitalClock  SampleTime=0.01
  Divide : Product  Inputs=*/
  Gain : Gain  Gain=pi
  Product : Product  RndMeth=Zero
  Trigonometric Function : Trigonometry
  constant : Constant
  experiment time step : Constant  Value=0.01  SampleTime=0
  enable : Outport
  wires:
  CAM_time_step/1 -> Divide/2
  Data Type Conversion/1 -> enable/1
  experiment time step/1 -> Add/2
  Add/1 -> Trigonometric Function/1
  Divide/1 -> Gain/1
  constant/1 -> Divide/1
  Product/1 -> Add/1
  Detect Change/1 -> Data Type Conversion/1
  Compare To Zero/1 -> Detect Change/1
  Trigonometric Function/1 -> Compare To Zero/1
  Gain/1 -> Product/2
  Digital Clock1/1 -> Product/1

== system EEBL_Scenario_03_cs/BMW_X5_1/vehicle CAM generator/set CAM signals ==
  CAM generation signal : Inport
  warning : Inport  Port=2
  messageID : Inport  Port=3
  vehicleID : Inport  Port=4
  vehicleType : Inport  Port=5
  publicVehicleType : Inport  Port=6
  lightBarInUse : Inport  Port=7
  sireneInUse : Inport  Port=8
  velocity : Inport  Port=9
  acceleration : Inport  Port=10
  yawRate : Inport  Port=11
  turnAdvice : Inport  Port=12
  trafficLightPriority : Inport  Port=13
  GPS_lat : Inport  Port=14
  GPS_long : Inport  Port=15
  GPS_alt : Inport  Port=16
  rotZ : Inport  Port=17
  Mux : Mux  Inputs=16
  Switch : Switch  Criteria=u2 > Threshold  Threshold=0.5
  Unit Delay : UnitDelay  SampleTime=-1
  CAM_signals : Outport
  wires:
  warning/1 -> Mux/1
  messageID/1 -> Mux/2
  vehicleID/1 -> Mux/3
  vehicleType/1 -> Mux/4
  publicVehicleType/1 -> Mux/5
  lightBarInUse/1 -> Mux/6
  sireneInUse/1 -> Mux/7
  velocity/1 -> Mux/8
  acceleration/1 -> Mux/9
  yawRate/1 -> Mux/10
  turnAdvice/1 -> Mux/11
  trafficLightPriority/1 -> Mux/12
  GPS_lat/1 -> Mux/13
  GPS_long/1 -> Mux/14
  GPS_alt/1 -> Mux/15
  rotZ/1 -> Mux/16
  CAM generation signal/1 -> Switch/2
  Mux/1 -> Switch/1
  Switch/1 -> Unit Delay/1, CAM_signals/1
  Unit Delay/1 -> Switch/3

== system EEBL_Scenario_03_cs/Nissan_Cabstar_1/Antenna_Rx_4_Demux/Reorder ==
  In : Inport
  Selector1 : Selector  InputPortWidth=InputPortWidth  IndexOptions=Index vector (dialog)  Indices=Elements  OutputSizes=1
  Out : Outport
  wires:
  Selector1/1 -> Out/1
  In/1 -> Selector1/1

== system EEBL_Scenario_03_cs/Nissan_Cabstar_1/Antenna_Rx_4_Demux/compas converter ==
  rotz [rad] : Inport
  cart2compas : Subsystem
  rad2deg : Gain  Gain=180/pi
  heading [deg] : Outport
  wires:
  rad2deg/1 -> cart2compas/1(Angle [deg])
  rotz [rad]/1 -> rad2deg/1
  cart2compas/1(heading [deg]) -> heading [deg]/1

== system EEBL_Scenario_03_cs/Nissan_Cabstar_1/SELF_Demux/compas converter ==
  rotz [rad] : Inport
  cart2compas : Subsystem
  rad2deg : Gain  Gain=180/pi
  heading [deg] : Outport
  wires:
  cart2compas/1(heading [deg]) -> heading [deg]/1
  rotz [rad]/1 -> rad2deg/1
  rad2deg/1 -> cart2compas/1(Angle [deg])

== system EEBL_Scenario_03_cs/Nissan_Cabstar_1/Trajectories/Traj2State1 ==
  Traj Org : Inport
  Offset : Inport  Port=2
  Add2 : Sum
  ApplyRotation : PreScanSimulinkLibrary/ApplyRotation  SystemSampleTime=-1
  ApplyRotation1 : PreScanSimulinkLibrary/ApplyRotation  SystemSampleTime=-1
  ApplyRotation2 : PreScanSimulinkLibrary/ApplyRotation  SystemSampleTime=-1
  Constant : Constant  Value=zeros(12,1)
  Mux : Mux  Inputs=6
  Mux1 : Mux  Inputs=2
  Mux{2,4..9} (7 alike) : Mux  Inputs=3
  Mux3 : Mux  Inputs=2
  Selector : Selector  InputPortWidth=6  IndexOptions=Index vector (dialog)  Indices=[4 5 6]  OutputSizes=1
  Selector1 : Selector  InputPortWidth=21  IndexOptions=Index vector (dialog)  Indices=[5]  OutputSizes=1
  Selector10 : Selector  InputPortWidth=21  IndexOptions=Index vector (dialog)  Indices=[2]  OutputSizes=1
  Selector11 : Selector  InputPortWidth=21  IndexOptions=Index vector (dialog)  Indices=[3]  OutputSizes=1
  Selector12 : Selector  InputPortWidth=21  IndexOptions=Index vector (dialog)  Indices=[1]  OutputSizes=1
  Selector13 : Selector  InputPortWidth=21  IndexOptions=Index vector (dialog)  Indices=[8]  OutputSizes=1
  Selector14 : Selector  InputPortWidth=21  IndexOptions=Index vector (dialog)  Indices=[9]  OutputSizes=1
  Selector15 : Selector  InputPortWidth=21  IndexOptions=Index vector (dialog)  Indices=[7]  OutputSizes=1
  Selector16 : Selector  InputPortWidth=21  IndexOptions=Index vector (dialog)  Indices=[14]  OutputSizes=1
  Selector17 : Selector  InputPortWidth=21  IndexOptions=Index vector (dialog)  Indices=[15]  OutputSizes=1
  Selector18 : Selector  InputPortWidth=21  IndexOptions=Index vector (dialog)  Indices=[13]  OutputSizes=1
  Selector19 : Selector  InputPortWidth=21  IndexOptions=Index vector (dialog)  Indices=[20]  OutputSizes=1
  Selector2 : Selector  InputPortWidth=21  IndexOptions=Index vector (dialog)  Indices=[6]  OutputSizes=1
  Selector20 : Selector  InputPortWidth=21  IndexOptions=Index vector (dialog)  Indices=[21]  OutputSizes=1
  Selector21 : Selector  InputPortWidth=21  IndexOptions=Index vector (dialog)  Indices=[19]  OutputSizes=1
  Selector3 : Selector  InputPortWidth=21  IndexOptions=Index vector (dialog)  Indices=[12]  OutputSizes=1
  Selector4 : Selector  InputPortWidth=21  IndexOptions=Index vector (dialog)  Indices=[17]  OutputSizes=1
  Selector5 : Selector  InputPortWidth=21  IndexOptions=Index vector (dialog)  Indices=[18]  OutputSizes=1
  Selector6 : Selector  InputPortWidth=21  IndexOptions=Index vector (dialog)  Indices=[16]  OutputSizes=1
  Selector7 : Selector  InputPortWidth=21  IndexOptions=Index vector (dialog)  Indices=[11]  OutputSizes=1
  Selector8 : Selector  InputPortWidth=21  IndexOptions=Index vector (dialog)  Indices=[10]  OutputSizes=1
  Selector9 : Selector  InputPortWidth=21  IndexOptions=Index vector (dialog)  Indices=[4]  OutputSizes=1
  Traj2State2 : Subsystem
  state : Outport
  wires:
  Mux9/1 -> ApplyRotation2/2, ApplyRotation1/2, ApplyRotation/2
  Selector20/1 -> Mux9/3
  Selector19/1 -> Mux9/2
  Selector21/1 -> Mux9/1
  Selector5/1 -> Mux8/3
  Selector4/1 -> Mux8/2
  Selector6/1 -> Mux8/1
  Mux8/1 -> Mux/6
  Mux6/1 -> ApplyRotation2/1
  Mux7/1 -> Mux/4
  ApplyRotation2/1 -> Mux/5
  Selector3/1 -> Mux7/3
  Selector7/1 -> Mux7/2
  Selector8/1 -> Mux7/1
  Mux4/1 -> Mux/2
  Mux5/1 -> ApplyRotation1/1
  ApplyRotation1/1 -> Mux/3
  Mux2/1 -> ApplyRotation/1
  ApplyRotation/1 -> Mux/1
  Selector2/1 -> Mux4/3
  Selector1/1 -> Mux4/2
  Selector9/1 -> Mux4/1
  Selector17/1 -> Mux6/3
  Selector16/1 -> Mux6/2
  Selector18/1 -> Mux6/1
  Selector14/1 -> Mux5/3
  Selector13/1 -> Mux5/2
  Selector15/1 -> Mux5/1
  Selector11/1 -> Mux2/3
  Selector10/1 -> Mux2/2
  Selector12/1 -> Mux2/1
  Mux3/1 -> Selector8/1, Selector7/1, Selector3/1, Selector18/1, Selector16/1, Selector17/1, Selector6/1, Selector20/1, Selector19/1, Selector21/1, Selector5/1, Selector4/1, Selector14/1, Selector13/1, Selector15/1, Selector2/1, Selector1/1, Selector9/1, Selector12/1, Selector10/1, Selector11/1
  Mux1/1 -> Add2/2
  Constant/1 -> Mux1/2
  Add2/1 -> Traj2State2/1(traj)
  Selector/1 -> Mux3/2
  Traj Org/1 -> Mux3/1
  Offset/1 -> Mux1/1, Selector/1
  Mux/1 -> Add2/1
  Traj2State2/1(state) -> state/1

== system EEBL_Scenario_03_cs/Nissan_Cabstar_1/Trajectories/Trajectory_3 ==
  From Workspace : FromWorkspace  VariableName=trajectory  SampleTime=TimeStep  OutputAfterFinalValue=Holding final value
  From Workspace1 : FromWorkspace  VariableName=trajectory  SampleTime=TimeStep  OutputAfterFinalValue=Setting to zero
  Mux : Mux  Inputs=2
  Selector1 : Selector  InputPortWidth=24  IndexOptions=Index vector (dialog)  Indices=[7:18]  OutputSizes=1
  Selector9 : Selector  InputPortWidth=24  IndexOptions=Index vector (dialog)  Indices=[1:6]  OutputSizes=1
  trajectory : Outport
  wires:
  Selector1/1 -> Mux/2
  Selector9/1 -> Mux/1
  Mux/1 -> trajectory/1
  From Workspace1/1 -> Selector1/1
  From Workspace/1 -> Selector9/1

== system EEBL_Scenario_03_cs/Nissan_Cabstar_1/vehicle CAM generator/CAM generation ==
  x [m] : Inport
  y [m] : Inport  Port=2
  z [m] : Inport  Port=3
  rotZ [deg] : Inport  Port=4
  velocity [m/s] : Inport  Port=5
  Enable : EnablePort  StatesWhenEnabling=reset  PropagateVarSize=During execution
  Add : Sum  Inputs=+-
  Data Store Memory : DataStoreMemory  DataStoreName=CAM_time
  Data Store Memory1 : DataStoreMemory  DataStoreName=CAM_velocity
  Data Store Memory2 : DataStoreMemory  DataStoreName=CAM_heading
  Data Store Memory3 : DataStoreMemory  DataStoreName=CAM_x
  Data Store Memory4 : DataStoreMemory  DataStoreName=CAM_y
  Data Store Memory5 : DataStoreMemory  DataStoreName=CAM_z
  Data Store Read : DataStoreRead  DataStoreName=CAM_time  SampleTime=0.01
  Digital Clock : DigitalClock  SampleTime=0.01
  Merge : Merge  Inputs=3
  if : If  IfExpression=u1 >= 1  ElseIfExpressions=u1 < 0.1
  maybe : Subsystem  TreatAsAtomicUnit=on
  no : Subsystem  TreatAsAtomicUnit=on
  yes : Subsystem  TreatAsAtomicUnit=on
  CAN generation signal : Outport  OutputWhenDisabled=reset  InitialOutput=0
  wires:
  Digital Clock/1 -> Add/1
  Data Store Read/1 -> Add/2
  Add/1 -> if/1
  if/1 -> yes/Action
  yes/1(Out1) -> Merge/1
  no/1(Out1) -> Merge/2
  if/2 -> no/Action
  if/3 -> maybe/Action
  Merge/1 -> CAN generation signal/1
  x [m]/1 -> maybe/1(x [m]), yes/1(x [m])
  y [m]/1 -> maybe/2(y [m]), yes/2(y [m])
  z [m]/1 -> maybe/3(z [m]), yes/3(z [m])
  rotZ [deg]/1 -> maybe/4(rotZ [deg]), yes/4(rotZ [deg])
  velocity [m/s]/1 -> maybe/5(velocity [m/s]), yes/5(velocity [m/s])
  maybe/1(Out1) -> Merge/3

== system EEBL_Scenario_03_cs/Nissan_Cabstar_1/vehicle CAM generator/Enabled Subsystem ==
  CAM_sig : Inport
  Enable : EnablePort  PropagateVarSize=During execution
  CAM_signals : Outport  OutputWhenDisabled=reset  InitialOutput=0
  wires:
  CAM_sig/1 -> CAM_signals/1

== system EEBL_Scenario_03_cs/Nissan_Cabstar_1/vehicle CAM generator/Subsystem ==
  In1 : Inport
  GPS_Noise_src : Inport  Port=2
  GPS Noise : Subsystem
  Sum2 : Sum  Inputs=|++
  Out1 : Outport
  wires:
  GPS Noise/1(GPS_Noise) -> Sum2/2
  In1/1 -> Sum2/1
  Sum2/1 -> Out1/1
  GPS_Noise_src/1 -> GPS Noise/1(GPS_Noise_src)

== system EEBL_Scenario_03_cs/Nissan_Cabstar_1/vehicle CAM generator/Subsystem1 ==
  In1 : Inport
  GPS_Noise_src : Inport  Port=2
  GPS Noise : Subsystem
  Sum2 : Sum  Inputs=|++
  Out1 : Outport
  wires:
  GPS_Noise_src/1 -> GPS Noise/1(GPS_Noise_src)
  Sum2/1 -> Out1/1
  In1/1 -> Sum2/1
  GPS Noise/1(GPS_Noise) -> Sum2/2

== system EEBL_Scenario_03_cs/Nissan_Cabstar_1/vehicle CAM generator/Subsystem2 ==
  In1 : Inport
  GPS_Noise_src : Inport  Port=2
  GPS Noise : Subsystem
  Sum2 : Sum  Inputs=|++
  Out1 : Outport
  wires:
  GPS Noise/1(GPS_Noise) -> Sum2/2
  In1/1 -> Sum2/1
  Sum2/1 -> Out1/1
  GPS_Noise_src/1 -> GPS Noise/1(GPS_Noise_src)

== system EEBL_Scenario_03_cs/Nissan_Cabstar_1/vehicle CAM generator/Subsystem3 ==
  In1 : Inport
  GPS_Noise_src : Inport  Port=2
  GPS Noise : Subsystem
  Sum2 : Sum  Inputs=|++
  Out1 : Outport
  wires:
  GPS_Noise_src/1 -> GPS Noise/1(GPS_Noise_src)
  Sum2/1 -> Out1/1
  In1/1 -> Sum2/1
  GPS Noise/1(GPS_Noise) -> Sum2/2

== system EEBL_Scenario_03_cs/Nissan_Cabstar_1/vehicle CAM generator/impulse generator ==
  CAM_time_step : Inport
  Add : Sum
  Compare To Zero : simulink/Logic and Bit Operations/Compare To Zero  SystemSampleTime=-1  relop=>  LogicOutDataTypeMode=boolean  ZeroCross=off
  Data Type Conversion : DataTypeConversion  OutDataTypeStr=boolean
  Detect Change : simulink/Logic and Bit Operations/Detect Change  SystemSampleTime=-1  vinit=0
  Digital Clock1 : DigitalClock  SampleTime=0.01
  Divide : Product  Inputs=*/
  Gain : Gain  Gain=pi
  Product : Product  RndMeth=Zero
  Trigonometric Function : Trigonometry
  constant : Constant
  experiment time step : Constant  Value=0.01  SampleTime=0
  enable : Outport
  wires:
  Digital Clock1/1 -> Product/1
  Gain/1 -> Product/2
  Trigonometric Function/1 -> Compare To Zero/1
  Compare To Zero/1 -> Detect Change/1
  Detect Change/1 -> Data Type Conversion/1
  Product/1 -> Add/1
  constant/1 -> Divide/1
  Divide/1 -> Gain/1
  Add/1 -> Trigonometric Function/1
  experiment time step/1 -> Add/2
  Data Type Conversion/1 -> enable/1
  CAM_time_step/1 -> Divide/2

== system EEBL_Scenario_03_cs/Nissan_Cabstar_1/vehicle CAM generator/impulse generator1 ==
  CAM_time_step : Inport
  Add : Sum
  Compare To Zero : simulink/Logic and Bit Operations/Compare To Zero  SystemSampleTime=-1  relop=>  LogicOutDataTypeMode=boolean  ZeroCross=off
  Data Type Conversion : DataTypeConversion  OutDataTypeStr=boolean
  Detect Change : simulink/Logic and Bit Operations/Detect Change  SystemSampleTime=-1  vinit=0
  Digital Clock1 : DigitalClock  SampleTime=0.01
  Divide : Product  Inputs=*/
  Gain : Gain  Gain=pi
  Product : Product  RndMeth=Zero
  Trigonometric Function : Trigonometry
  constant : Constant
  experiment time step : Constant  Value=0.01  SampleTime=0
  enable : Outport
  wires:
  CAM_time_step/1 -> Divide/2
  Data Type Conversion/1 -> enable/1
  experiment time step/1 -> Add/2
  Add/1 -> Trigonometric Function/1
  Divide/1 -> Gain/1
  constant/1 -> Divide/1
  Product/1 -> Add/1
  Detect Change/1 -> Data Type Conversion/1
  Compare To Zero/1 -> Detect Change/1
  Trigonometric Function/1 -> Compare To Zero/1
  Gain/1 -> Product/2
  Digital Clock1/1 -> Product/1

== system EEBL_Scenario_03_cs/Nissan_Cabstar_1/vehicle CAM generator/set CAM signals ==
  CAM generation signal : Inport
  warning : Inport  Port=2
  messageID : Inport  Port=3
  vehicleID : Inport  Port=4
  vehicleType : Inport  Port=5
  publicVehicleType : Inport  Port=6
  lightBarInUse : Inport  Port=7
  sireneInUse : Inport  Port=8
  velocity : Inport  Port=9
  acceleration : Inport  Port=10
  yawRate : Inport  Port=11
  turnAdvice : Inport  Port=12
  trafficLightPriority : Inport  Port=13
  GPS_lat : Inport  Port=14
  GPS_long : Inport  Port=15
  GPS_alt : Inport  Port=16
  rotZ : Inport  Port=17
  Mux : Mux  Inputs=16
  Switch : Switch  Criteria=u2 > Threshold  Threshold=0.5
  Unit Delay : UnitDelay  SampleTime=-1
  CAM_signals : Outport
  wires:
  warning/1 -> Mux/1
  messageID/1 -> Mux/2
  vehicleID/1 -> Mux/3
  vehicleType/1 -> Mux/4
  publicVehicleType/1 -> Mux/5
  lightBarInUse/1 -> Mux/6
  sireneInUse/1 -> Mux/7
  velocity/1 -> Mux/8
  acceleration/1 -> Mux/9
  yawRate/1 -> Mux/10
  turnAdvice/1 -> Mux/11
  trafficLightPriority/1 -> Mux/12
  GPS_lat/1 -> Mux/13
  GPS_long/1 -> Mux/14
  GPS_alt/1 -> Mux/15
  rotZ/1 -> Mux/16
  CAM generation signal/1 -> Switch/2
  Mux/1 -> Switch/1
  Switch/1 -> Unit Delay/1, CAM_signals/1
  Unit Delay/1 -> Switch/3

== system EEBL_Scenario_03_cs/RectangularBox_1/Antenna_Rx_2_Demux/Reorder ==
  In : Inport
  Selector1 : Selector  InputPortWidth=InputPortWidth  IndexOptions=Index vector (dialog)  Indices=Elements  OutputSizes=1
  Out : Outport
  wires:
  Selector1/1 -> Out/1
  In/1 -> Selector1/1

== system EEBL_Scenario_03_cs/RectangularBox_1/Antenna_Rx_2_Demux/compas converter ==
  rotz [rad] : Inport
  cart2compas : Subsystem
  rad2deg : Gain  Gain=180/pi
  heading [deg] : Outport
  wires:
  rad2deg/1 -> cart2compas/1(Angle [deg])
  rotz [rad]/1 -> rad2deg/1
  cart2compas/1(heading [deg]) -> heading [deg]/1
